simulink model "req16"  (R2019a)
settings: Solver=FixedStepAuto  StartTime=0.0  StopTime=1000  FixedStep=0.01  RelTol=1e-3
libraries: simulink x10
settings Model: Creator=e40014285  LastModifiedBy=e40014285
settings ConfigComp: CovScope=ReferencedModels  CovHTMLOptions=-sRT=1 -sVT=0 -aTS=1 -bRG=1 -bTC=1 -hTR=0 -nFC=0 -nFD=1 -scm=1 -bcm=1 -xEv=0 -xEM=0  CovHtmlReporting=on  CovCumulativeReport=on  DVMaxProcessTime=6000  DVModelCoverageObjectives=EnhancedMCDC  DVTestSuiteOptimization=Auto  DVDetectOutOfBounds=on  DVReportPDFFormat=on  DVRebuildModelRepresentation=Always

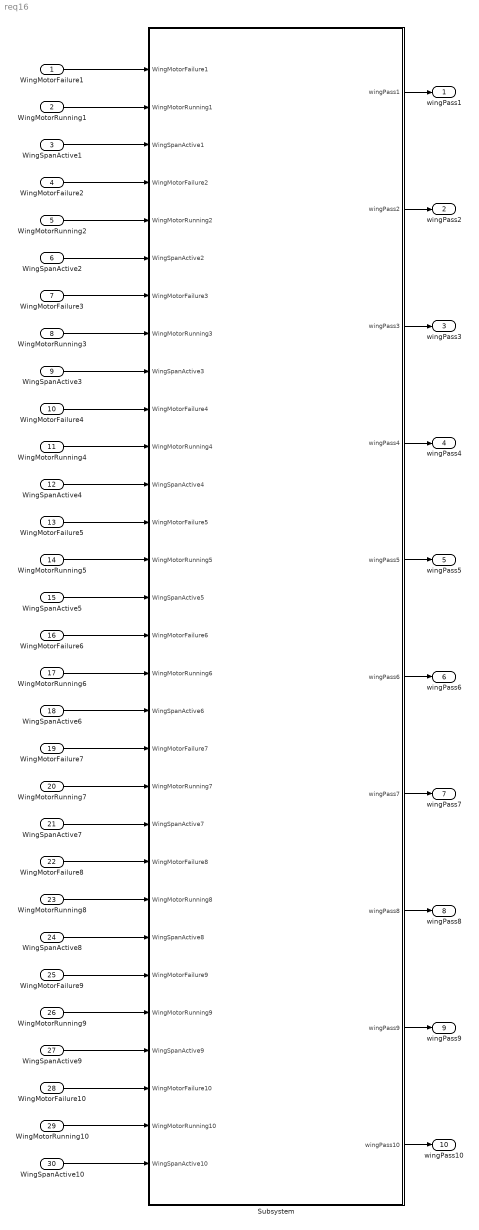
== system req16 ==
  WingMotorFailure1 : Inport
  WingMotorRunning1 : Inport  Port=2
  WingSpanActive1 : Inport  Port=3
  WingMotorFailure2 : Inport  Port=4
  WingMotorRunning2 : Inport  Port=5
  WingSpanActive2 : Inport  Port=6
  WingMotorFailure3 : Inport  Port=7
  WingMotorRunning3 : Inport  Port=8
  WingSpanActive3 : Inport  Port=9
  WingMotorFailure4 : Inport  Port=10
  WingMotorRunning4 : Inport  Port=11
  WingSpanActive4 : Inport  Port=12
  WingMotorFailure5 : Inport  Port=13
  WingMotorRunning5 : Inport  Port=14
  WingSpanActive5 : Inport  Port=15
  WingMotorFailure6 : Inport  Port=16
  WingMotorRunning6 : Inport  Port=17
  WingSpanActive6 : Inport  Port=18
  WingMotorFailure7 : Inport  Port=19
  WingMotorRunning7 : Inport  Port=20
  WingSpanActive7 : Inport  Port=21
  WingMotorFailure8 : Inport  Port=22
  WingMotorRunning8 : Inport  Port=23
  WingSpanActive8 : Inport  Port=24
  WingMotorFailure9 : Inport  Port=25
  WingMotorRunning9 : Inport  Port=26
  WingSpanActive9 : Inport  Port=27
  WingMotorFailure10 : Inport  Port=28
  WingMotorRunning10 : Inport  Port=29
  WingSpanActive10 : Inport  Port=30
  Subsystem : Subsystem
  wingPass1 : Outport
  wingPass2 : Outport  Port=2
  wingPass3 : Outport  Port=3
  wingPass4 : Outport  Port=4
  wingPass5 : Outport  Port=5
  wingPass6 : Outport  Port=6
  wingPass7 : Outport  Port=7
  wingPass8 : Outport  Port=8
  wingPass9 : Outport  Port=9
  wingPass10 : Outport  Port=10
  wires:
  Subsystem/2(wingPass2) -> wingPass2/1
  Subsystem/7(wingPass7) -> wingPass7/1
  Subsystem/3(wingPass3) -> wingPass3/1
  WingSpanActive10/1 -> Subsystem/30(WingSpanActive10)
  Subsystem/6(wingPass6) -> wingPass6/1
  Subsystem/8(wingPass8) -> wingPass8/1
  Subsystem/10(wingPass10) -> wingPass10/1
  Subsystem/4(wingPass4) -> wingPass4/1
  Subsystem/5(wingPass5) -> wingPass5/1
  Subsystem/9(wingPass9) -> wingPass9/1
  WingMotorFailure5/1 -> Subsystem/13(WingMotorFailure5)
  Subsystem/1(wingPass1) -> wingPass1/1
  WingMotorRunning10/1 -> Subsystem/29(WingMotorRunning10)
  WingSpanActive8/1 -> Subsystem/24(WingSpanActive8)
  WingMotorFailure10/1 -> Subsystem/28(WingMotorFailure10)
  WingSpanActive9/1 -> Subsystem/27(WingSpanActive9)
  WingMotorRunning9/1 -> Subsystem/26(WingMotorRunning9)
  WingMotorFailure9/1 -> Subsystem/25(WingMotorFailure9)
  WingMotorRunning8/1 -> Subsystem/23(WingMotorRunning8)
  WingMotorFailure8/1 -> Subsystem/22(WingMotorFailure8)
  WingSpanActive7/1 -> Subsystem/21(WingSpanActive7)
  WingSpanActive4/1 -> Subsystem/12(WingSpanActive4)
  WingMotorRunning7/1 -> Subsystem/20(WingMotorRunning7)
  WingMotorFailure7/1 -> Subsystem/19(WingMotorFailure7)
  WingSpanActive6/1 -> Subsystem/18(WingSpanActive6)
  WingMotorRunning3/1 -> Subsystem/8(WingMotorRunning3)
  WingMotorRunning6/1 -> Subsystem/17(WingMotorRunning6)
  WingMotorFailure6/1 -> Subsystem/16(WingMotorFailure6)
  WingSpanActive1/1 -> Subsystem/3(WingSpanActive1)
  WingSpanActive2/1 -> Subsystem/6(WingSpanActive2)
  WingSpanActive5/1 -> Subsystem/15(WingSpanActive5)
  WingMotorRunning5/1 -> Subsystem/14(WingMotorRunning5)
  WingSpanActive3/1 -> Subsystem/9(WingSpanActive3)
  WingMotorFailure3/1 -> Subsystem/7(WingMotorFailure3)
  WingMotorRunning4/1 -> Subsystem/11(WingMotorRunning4)
  WingMotorFailure4/1 -> Subsystem/10(WingMotorFailure4)
  WingMotorFailure2/1 -> Subsystem/4(WingMotorFailure2)
  WingMotorRunning2/1 -> Subsystem/5(WingMotorRunning2)
  WingMotorRunning1/1 -> Subsystem/2(WingMotorRunning1)
  WingMotorFailure1/1 -> Subsystem/1(WingMotorFailure1)

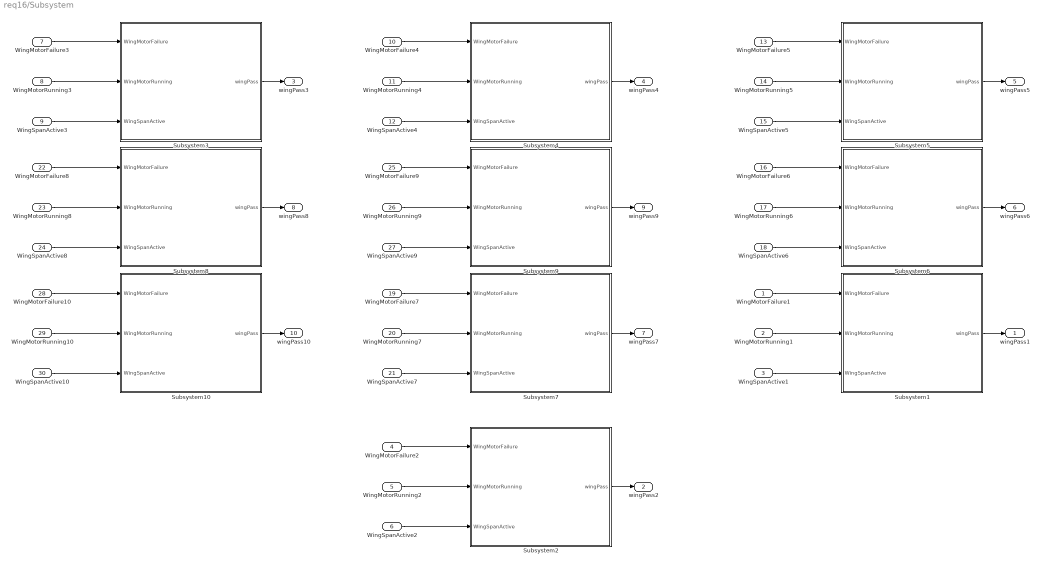
== system req16/Subsystem ==
  WingMotorFailure1 : Inport
  WingMotorRunning1 : Inport  Port=2
  WingSpanActive1 : Inport  Port=3
  WingMotorFailure2 : Inport  Port=4
  WingMotorRunning2 : Inport  Port=5
  WingSpanActive2 : Inport  Port=6
  WingMotorFailure3 : Inport  Port=7
  WingMotorRunning3 : Inport  Port=8
  WingSpanActive3 : Inport  Port=9
  WingMotorFailure4 : Inport  Port=10
  WingMotorRunning4 : Inport  Port=11
  WingSpanActive4 : Inport  Port=12
  WingMotorFailure5 : Inport  Port=13
  WingMotorRunning5 : Inport  Port=14
  WingSpanActive5 : Inport  Port=15
  WingMotorFailure6 : Inport  Port=16
  WingMotorRunning6 : Inport  Port=17
  WingSpanActive6 : Inport  Port=18
  WingMotorFailure7 : Inport  Port=19
  WingMotorRunning7 : Inport  Port=20
  WingSpanActive7 : Inport  Port=21
  WingMotorFailure8 : Inport  Port=22
  WingMotorRunning8 : Inport  Port=23
  WingSpanActive8 : Inport  Port=24
  WingMotorFailure9 : Inport  Port=25
  WingMotorRunning9 : Inport  Port=26
  WingSpanActive9 : Inport  Port=27
  WingMotorFailure10 : Inport  Port=28
  WingMotorRunning10 : Inport  Port=29
  WingSpanActive10 : Inport  Port=30
  Subsystem1 : Subsystem
  Subsystem10 : Subsystem
  Subsystem2 : Subsystem
  Subsystem3 : Subsystem
  Subsystem4 : Subsystem
  Subsystem5 : Subsystem
  Subsystem6 : Subsystem
  Subsystem7 : Subsystem
  Subsystem8 : Subsystem
  Subsystem9 : Subsystem
  wingPass1 : Outport
  wingPass2 : Outport  Port=2
  wingPass3 : Outport  Port=3
  wingPass4 : Outport  Port=4
  wingPass5 : Outport  Port=5
  wingPass6 : Outport  Port=6
  wingPass7 : Outport  Port=7
  wingPass8 : Outport  Port=8
  wingPass9 : Outport  Port=9
  wingPass10 : Outport  Port=10
  wires:
  WingSpanActive6/1 -> Subsystem6/3(WingSpanActive)
  WingMotorFailure10/1 -> Subsystem10/1(WingMotorFailure)
  WingMotorFailure9/1 -> Subsystem9/1(WingMotorFailure)
  WingMotorRunning7/1 -> Subsystem7/2(WingMotorRunning)
  WingSpanActive3/1 -> Subsystem3/3(WingSpanActive)
  WingMotorRunning5/1 -> Subsystem5/2(WingMotorRunning)
  WingSpanActive7/1 -> Subsystem7/3(WingSpanActive)
  WingSpanActive10/1 -> Subsystem10/3(WingSpanActive)
  WingMotorFailure3/1 -> Subsystem3/1(WingMotorFailure)
  WingSpanActive9/1 -> Subsystem9/3(WingSpanActive)
  Subsystem4/1(wingPass) -> wingPass4/1
  WingMotorFailure2/1 -> Subsystem2/1(WingMotorFailure)
  WingSpanActive8/1 -> Subsystem8/3(WingSpanActive)
  Subsystem3/1(wingPass) -> wingPass3/1
  WingMotorRunning1/1 -> Subsystem1/2(WingMotorRunning)
  WingMotorFailure8/1 -> Subsystem8/1(WingMotorFailure)
  WingMotorFailure1/1 -> Subsystem1/1(WingMotorFailure)
  WingMotorRunning4/1 -> Subsystem4/2(WingMotorRunning)
  WingSpanActive4/1 -> Subsystem4/3(WingSpanActive)
  WingMotorRunning8/1 -> Subsystem8/2(WingMotorRunning)
  WingMotorRunning3/1 -> Subsystem3/2(WingMotorRunning)
  WingMotorRunning9/1 -> Subsystem9/2(WingMotorRunning)
  WingMotorFailure7/1 -> Subsystem7/1(WingMotorFailure)
  WingSpanActive5/1 -> Subsystem5/3(WingSpanActive)
  WingMotorRunning10/1 -> Subsystem10/2(WingMotorRunning)
  WingMotorFailure6/1 -> Subsystem6/1(WingMotorFailure)
  WingMotorFailure4/1 -> Subsystem4/1(WingMotorFailure)
  WingSpanActive1/1 -> Subsystem1/3(WingSpanActive)
  WingMotorFailure5/1 -> Subsystem5/1(WingMotorFailure)
  WingMotorRunning6/1 -> Subsystem6/2(WingMotorRunning)
  WingSpanActive2/1 -> Subsystem2/3(WingSpanActive)
  WingMotorRunning2/1 -> Subsystem2/2(WingMotorRunning)
  Subsystem2/1(wingPass) -> wingPass2/1
  Subsystem9/1(wingPass) -> wingPass9/1
  Subsystem1/1(wingPass) -> wingPass1/1
  Subsystem8/1(wingPass) -> wingPass8/1
  Subsystem7/1(wingPass) -> wingPass7/1
  Subsystem5/1(wingPass) -> wingPass5/1
  Subsystem6/1(wingPass) -> wingPass6/1
  Subsystem10/1(wingPass) -> wingPass10/1

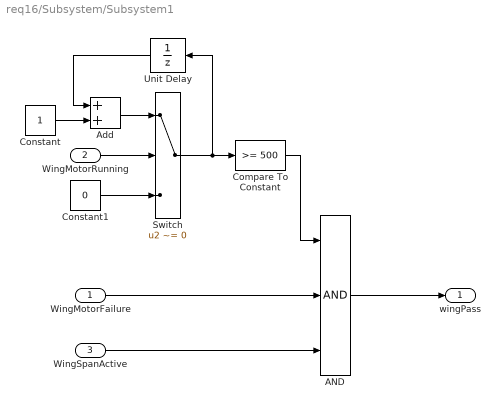
== system req16/Subsystem/Subsystem1 ==
  WingMotorFailure : Inport
  WingMotorRunning : Inport  Port=2
  WingSpanActive : Inport  Port=3
  AND : Logic  Inputs=3  AllPortsSameDT=off  OutDataTypeStr=boolean
  Add : Sum
  Compare To Constant : simulink/Logic and Bit Operations/Compare To Constant  relop=>=  const=500  OutDataTypeStr=boolean
  Constant : Constant
  Constant1 : Constant  Value=0
  Switch : Switch  Criteria=u2 ~= 0
  Unit Delay : UnitDelay  SampleTime=-1  HasFrameUpgradeWarning=on
  wingPass : Outport
  wires:
  WingMotorFailure/1 -> AND/2
  Unit Delay/1 -> Add/1
  Add/1 -> Switch/1
  WingMotorRunning/1 -> Switch/2
  WingSpanActive/1 -> AND/3
  AND/1 -> wingPass/1
  Constant1/1 -> Switch/3
  Constant/1 -> Add/2
  Switch/1 -> Compare To Constant/1, Unit Delay/1
  Compare To Constant/1 -> AND/1

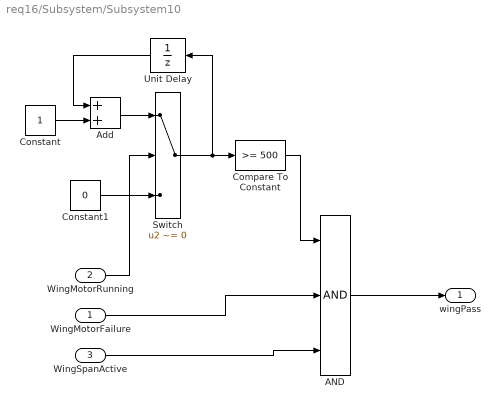
== system req16/Subsystem/Subsystem10 ==
  WingMotorFailure : Inport
  WingMotorRunning : Inport  Port=2
  WingSpanActive : Inport  Port=3
  AND : Logic  Inputs=3  AllPortsSameDT=off  OutDataTypeStr=boolean
  Add : Sum
  Compare To Constant : simulink/Logic and Bit Operations/Compare To Constant  relop=>=  const=500  OutDataTypeStr=boolean
  Constant : Constant
  Constant1 : Constant  Value=0
  Switch : Switch  Criteria=u2 ~= 0
  Unit Delay : UnitDelay  SampleTime=-1  HasFrameUpgradeWarning=on
  wingPass : Outport
  wires:
  WingMotorFailure/1 -> AND/2
  Unit Delay/1 -> Add/1
  Add/1 -> Switch/1
  WingMotorRunning/1 -> Switch/2
  WingSpanActive/1 -> AND/3
  AND/1 -> wingPass/1
  Constant1/1 -> Switch/3
  Constant/1 -> Add/2
  Switch/1 -> Compare To Constant/1, Unit Delay/1
  Compare To Constant/1 -> AND/1

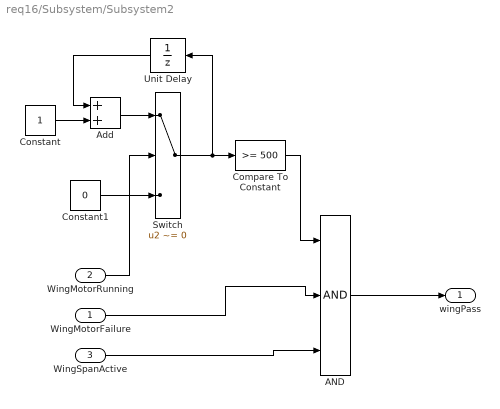
== system req16/Subsystem/Subsystem2 ==
  WingMotorFailure : Inport
  WingMotorRunning : Inport  Port=2
  WingSpanActive : Inport  Port=3
  AND : Logic  Inputs=3  AllPortsSameDT=off  OutDataTypeStr=boolean
  Add : Sum
  Compare To Constant : simulink/Logic and Bit Operations/Compare To Constant  relop=>=  const=500  OutDataTypeStr=boolean
  Constant : Constant
  Constant1 : Constant  Value=0
  Switch : Switch  Criteria=u2 ~= 0
  Unit Delay : UnitDelay  SampleTime=-1  HasFrameUpgradeWarning=on
  wingPass : Outport
  wires:
  WingMotorFailure/1 -> AND/2
  Unit Delay/1 -> Add/1
  Add/1 -> Switch/1
  WingMotorRunning/1 -> Switch/2
  WingSpanActive/1 -> AND/3
  AND/1 -> wingPass/1
  Constant1/1 -> Switch/3
  Constant/1 -> Add/2
  Switch/1 -> Compare To Constant/1, Unit Delay/1
  Compare To Constant/1 -> AND/1

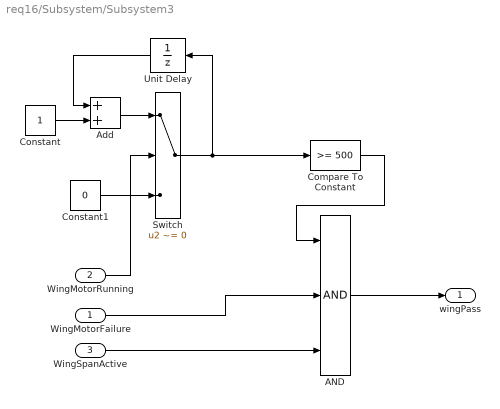
== system req16/Subsystem/Subsystem3 ==
  WingMotorFailure : Inport
  WingMotorRunning : Inport  Port=2
  WingSpanActive : Inport  Port=3
  AND : Logic  Inputs=3  AllPortsSameDT=off  OutDataTypeStr=boolean
  Add : Sum
  Compare To Constant : simulink/Logic and Bit Operations/Compare To Constant  relop=>=  const=500  OutDataTypeStr=boolean
  Constant : Constant
  Constant1 : Constant  Value=0
  Switch : Switch  Criteria=u2 ~= 0
  Unit Delay : UnitDelay  SampleTime=-1  HasFrameUpgradeWarning=on
  wingPass : Outport
  wires:
  WingMotorFailure/1 -> AND/2
  Unit Delay/1 -> Add/1
  Add/1 -> Switch/1
  WingMotorRunning/1 -> Switch/2
  WingSpanActive/1 -> AND/3
  AND/1 -> wingPass/1
  Constant1/1 -> Switch/3
  Constant/1 -> Add/2
  Switch/1 -> Compare To Constant/1, Unit Delay/1
  Compare To Constant/1 -> AND/1

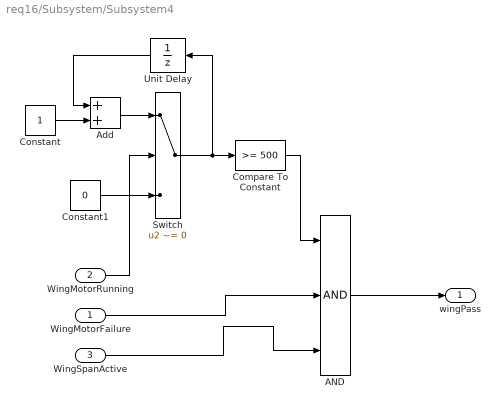
== system req16/Subsystem/Subsystem4 ==
  WingMotorFailure : Inport
  WingMotorRunning : Inport  Port=2
  WingSpanActive : Inport  Port=3
  AND : Logic  Inputs=3  AllPortsSameDT=off  OutDataTypeStr=boolean
  Add : Sum
  Compare To Constant : simulink/Logic and Bit Operations/Compare To Constant  relop=>=  const=500  OutDataTypeStr=boolean
  Constant : Constant
  Constant1 : Constant  Value=0
  Switch : Switch  Criteria=u2 ~= 0
  Unit Delay : UnitDelay  SampleTime=-1  HasFrameUpgradeWarning=on
  wingPass : Outport
  wires:
  WingMotorFailure/1 -> AND/2
  Unit Delay/1 -> Add/1
  Add/1 -> Switch/1
  WingMotorRunning/1 -> Switch/2
  WingSpanActive/1 -> AND/3
  AND/1 -> wingPass/1
  Constant1/1 -> Switch/3
  Constant/1 -> Add/2
  Switch/1 -> Compare To Constant/1, Unit Delay/1
  Compare To Constant/1 -> AND/1

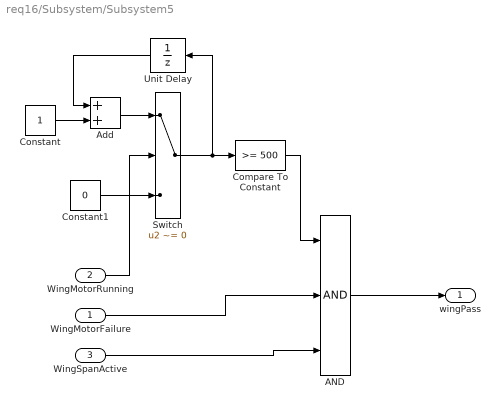
== system req16/Subsystem/Subsystem5 ==
  WingMotorFailure : Inport
  WingMotorRunning : Inport  Port=2
  WingSpanActive : Inport  Port=3
  AND : Logic  Inputs=3  AllPortsSameDT=off  OutDataTypeStr=boolean
  Add : Sum
  Compare To Constant : simulink/Logic and Bit Operations/Compare To Constant  relop=>=  const=500  OutDataTypeStr=boolean
  Constant : Constant
  Constant1 : Constant  Value=0
  Switch : Switch  Criteria=u2 ~= 0
  Unit Delay : UnitDelay  SampleTime=-1  HasFrameUpgradeWarning=on
  wingPass : Outport
  wires:
  WingMotorFailure/1 -> AND/2
  Unit Delay/1 -> Add/1
  Add/1 -> Switch/1
  WingMotorRunning/1 -> Switch/2
  WingSpanActive/1 -> AND/3
  AND/1 -> wingPass/1
  Constant1/1 -> Switch/3
  Constant/1 -> Add/2
  Switch/1 -> Compare To Constant/1, Unit Delay/1
  Compare To Constant/1 -> AND/1

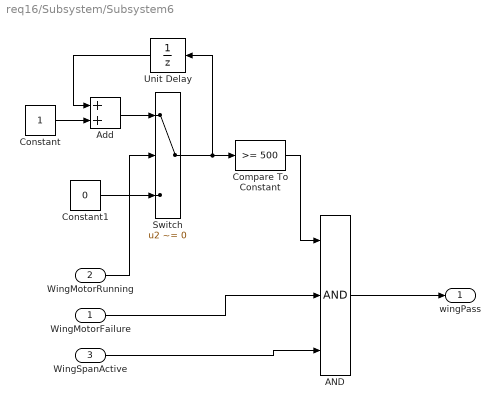
== system req16/Subsystem/Subsystem6 ==
  WingMotorFailure : Inport
  WingMotorRunning : Inport  Port=2
  WingSpanActive : Inport  Port=3
  AND : Logic  Inputs=3  AllPortsSameDT=off  OutDataTypeStr=boolean
  Add : Sum
  Compare To Constant : simulink/Logic and Bit Operations/Compare To Constant  relop=>=  const=500  OutDataTypeStr=boolean
  Constant : Constant
  Constant1 : Constant  Value=0
  Switch : Switch  Criteria=u2 ~= 0
  Unit Delay : UnitDelay  SampleTime=-1  HasFrameUpgradeWarning=on
  wingPass : Outport
  wires:
  WingMotorFailure/1 -> AND/2
  Unit Delay/1 -> Add/1
  Add/1 -> Switch/1
  WingMotorRunning/1 -> Switch/2
  WingSpanActive/1 -> AND/3
  AND/1 -> wingPass/1
  Constant1/1 -> Switch/3
  Constant/1 -> Add/2
  Switch/1 -> Compare To Constant/1, Unit Delay/1
  Compare To Constant/1 -> AND/1

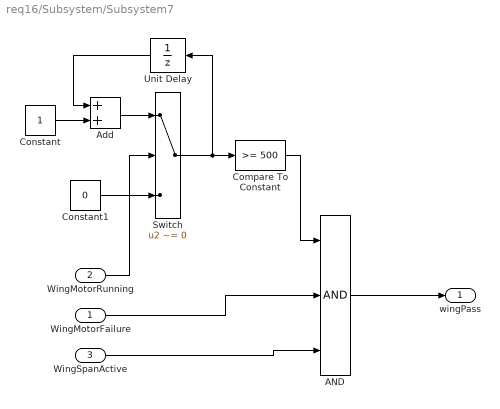
== system req16/Subsystem/Subsystem7 ==
  WingMotorFailure : Inport
  WingMotorRunning : Inport  Port=2
  WingSpanActive : Inport  Port=3
  AND : Logic  Inputs=3  AllPortsSameDT=off  OutDataTypeStr=boolean
  Add : Sum
  Compare To Constant : simulink/Logic and Bit Operations/Compare To Constant  relop=>=  const=500  OutDataTypeStr=boolean
  Constant : Constant
  Constant1 : Constant  Value=0
  Switch : Switch  Criteria=u2 ~= 0
  Unit Delay : UnitDelay  SampleTime=-1  HasFrameUpgradeWarning=on
  wingPass : Outport
  wires:
  WingMotorFailure/1 -> AND/2
  Unit Delay/1 -> Add/1
  Add/1 -> Switch/1
  WingMotorRunning/1 -> Switch/2
  WingSpanActive/1 -> AND/3
  AND/1 -> wingPass/1
  Constant1/1 -> Switch/3
  Constant/1 -> Add/2
  Switch/1 -> Compare To Constant/1, Unit Delay/1
  Compare To Constant/1 -> AND/1

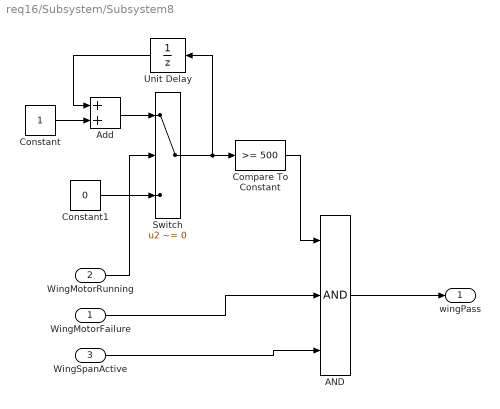
== system req16/Subsystem/Subsystem8 ==
  WingMotorFailure : Inport
  WingMotorRunning : Inport  Port=2
  WingSpanActive : Inport  Port=3
  AND : Logic  Inputs=3  AllPortsSameDT=off  OutDataTypeStr=boolean
  Add : Sum
  Compare To Constant : simulink/Logic and Bit Operations/Compare To Constant  relop=>=  const=500  OutDataTypeStr=boolean
  Constant : Constant
  Constant1 : Constant  Value=0
  Switch : Switch  Criteria=u2 ~= 0
  Unit Delay : UnitDelay  SampleTime=-1  HasFrameUpgradeWarning=on
  wingPass : Outport
  wires:
  WingMotorFailure/1 -> AND/2
  Unit Delay/1 -> Add/1
  Add/1 -> Switch/1
  WingMotorRunning/1 -> Switch/2
  WingSpanActive/1 -> AND/3
  AND/1 -> wingPass/1
  Constant1/1 -> Switch/3
  Constant/1 -> Add/2
  Switch/1 -> Compare To Constant/1, Unit Delay/1
  Compare To Constant/1 -> AND/1

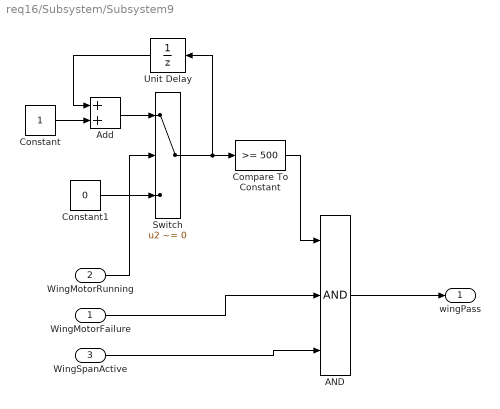
== system req16/Subsystem/Subsystem9 ==
  WingMotorFailure : Inport
  WingMotorRunning : Inport  Port=2
  WingSpanActive : Inport  Port=3
  AND : Logic  Inputs=3  AllPortsSameDT=off  OutDataTypeStr=boolean
  Add : Sum
  Compare To Constant : simulink/Logic and Bit Operations/Compare To Constant  relop=>=  const=500  OutDataTypeStr=boolean
  Constant : Constant
  Constant1 : Constant  Value=0
  Switch : Switch  Criteria=u2 ~= 0
  Unit Delay : UnitDelay  SampleTime=-1  HasFrameUpgradeWarning=on
  wingPass : Outport
  wires:
  WingMotorFailure/1 -> AND/2
  Unit Delay/1 -> Add/1
  Add/1 -> Switch/1
  WingMotorRunning/1 -> Switch/2
  WingSpanActive/1 -> AND/3
  AND/1 -> wingPass/1
  Constant1/1 -> Switch/3
  Constant/1 -> Add/2
  Switch/1 -> Compare To Constant/1, Unit Delay/1
  Compare To Constant/1 -> AND/1
